simulink model "OpenLoopTest_animacion"  (R2023a)
settings: Solver=VariableStepAuto  StartTime=0.0  StopTime=50  RelTol=1e-3
model workspace (MAT data in the model file):
  A = 0.000165129963854
  B = 2.18020469989e-05
  I = [0.0336109715  0  0; 0  0.0308250765  0; 0  0  0.0271714972]
  Iw = [7.613e-05  0  0; 0  7.613e-05  0; 0  0  7.613e-05]
  J = 7.613e-05
  Ke = 0.00852615766564
  Kt = 0.00855
  L = 0.585
  La = 0.000222
  Ra = 3.36
  T_ext = 6.85e-07
  T_max = 7.7501
  T_max_mgt = -0.018432
  coil_longitude = 7.92
  dia_coil = 2
  dia_core = 0.77
  dia_wire = 0.03
  l = 0.0792
  mu_0 = 1.25663706212e-06
  mu_r = 200000
  n = 33.4123983836
  n_cal = 5412
  n_layers = 20.5
  s = tf
  s.IOSize_ = [1 1]
  s.Data_ = ltipack.tfdata
  s.Data_.num = {[1 0]}
  s.Data_.den = {[0 1]}
  s.Data_.Delay.Input = 0
  s.Data_.Delay.Output = 0
  s.Data_.Delay.IO = 0
  s.Data_.Ts = 0
  sys = tf
  sys.IOSize_ = [1 1]
  sys.Data_ = ltipack.tfdata
  sys.Data_.num = {[0 6.509115e-07 1.86407501841e-07]}
  sys.Data_.den = {[1.690086e-08 0.000255801640054 0.000146153525957]}
  sys.Data_.Delay.Input = 0
  sys.Data_.Delay.Output = 0
  sys.Data_.Delay.IO = 0
  sys.Data_.Ts = 0
  turns_per_layer = 264
  voltaje = 9
libraries: simulink_extras x6, aerolibutil x2, vrlib x1, shared6dofsys x1
settings Model: Creator=Personal  LastModifiedBy=Personal
settings OptimizationCC: ReuseModelBlockBuffer=off

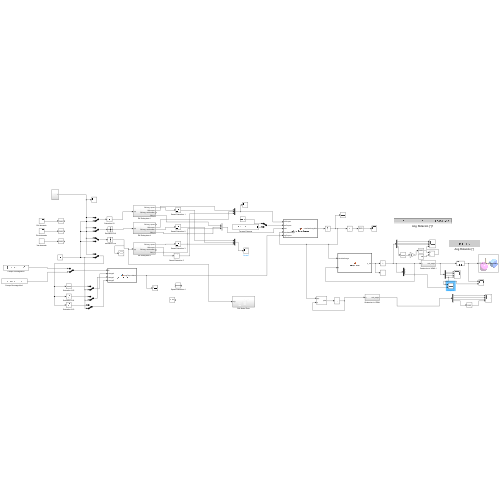
[thumbnail: Simulink's stored preview of the top-level diagram]
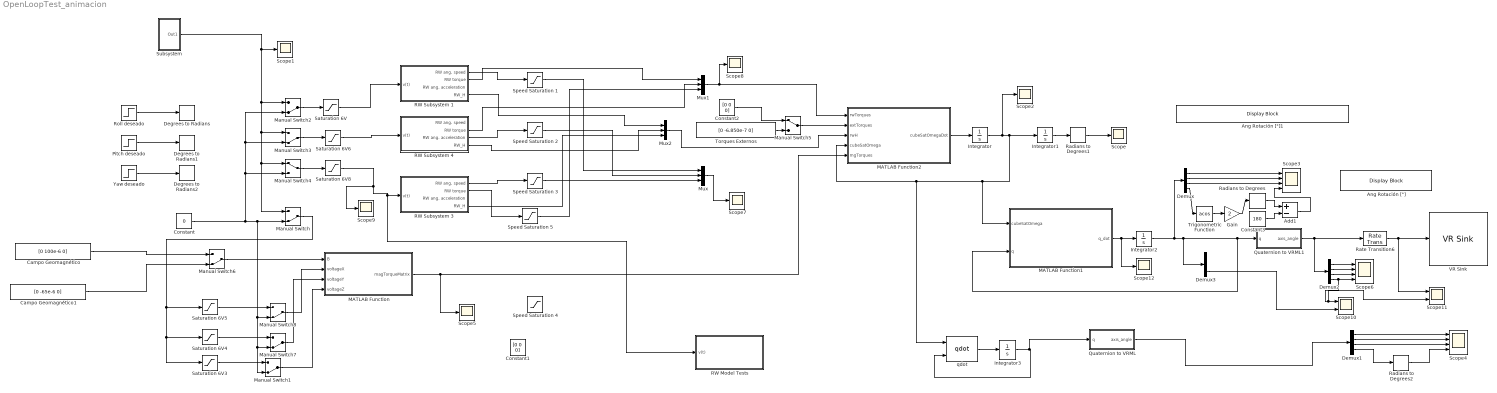
== system OpenLoopTest_animacion ==
  Add1 : Sum  Inputs=+-
  Ang Rotación [°] : DisplayBlock  LabelPosition=Hide  Transparency=1
  Ang Rotación [°]1 : DisplayBlock  LabelPosition=Hide  Transparency=1
  Campo Geomagnético : Constant  Value=[0 100e-6 0]
  Campo Geomagnético1 : Constant  Value=[0 -65e-6 0]
  Constant : Constant  Value=0
  Constant1 : Constant  Value=[0 0 0]
  Constant2 : Constant  Value=[0 0 0]
  Constant3 : Constant  Value=180
  Degrees to Radians : simulink_extras/Transformations/Degrees to Radians
  Degrees to Radians1 : simulink_extras/Transformations/Degrees to Radians
  Degrees to Radians2 : simulink_extras/Transformations/Degrees to Radians
  Demux{,1..3} (4 alike) : Demux
  Gain : Gain  Gain=2
  Integrator : Integrator  InitialCondition=[0 0 0]
  Integrator1 : Integrator  InitialCondition=[0 0 0]
  Integrator2 : Integrator  InitialCondition=[0 0 1 0]
  Integrator3 : Integrator  InitialCondition=[0 1 0 0]
  MATLAB Function : MATLAB Function  TreatAsAtomicUnit=on
  MATLAB Function1 : MATLAB Function  TreatAsAtomicUnit=on
  MATLAB Function2 : MATLAB Function  TreatAsAtomicUnit=on
  Manual Switch{,1..3,6..8} (7 alike) : ManualSwitch  CurrentSetting=0
  Manual Switch4 : ManualSwitch
  Manual Switch5 : ManualSwitch
  Mux : Mux  Inputs=3
  Mux1 : Mux  Inputs=3
  Mux2 : Mux  Inputs=3
  Pitch deseado : Step  Time=2  After=0  SampleTime=0
  Quaternion to VRML : Subsystem
  Quaternion to VRML1 : Subsystem
  RW Model Tests : Subsystem
  RW Subsystem 1 : Subsystem
  RW Subsystem 3 : Subsystem
  RW Subsystem 4 : Subsystem
  Radians to Degrees : simulink_extras/Transformations/Radians to Degrees
  Radians to Degrees1 : simulink_extras/Transformations/Radians to Degrees
  Radians to Degrees2 : simulink_extras/Transformations/Radians to Degrees
  Rate Transition6 : RateTransition
  Roll deseado : Step  Time=2  After=90  SampleTime=0
  Saturation 6V : Saturate  UpperLimit=5  LowerLimit=-5
  Saturation 6V3 : Saturate  UpperLimit=6  LowerLimit=-6
  Saturation 6V4 : Saturate  UpperLimit=2  LowerLimit=-6
  Saturation 6V5 : Saturate  UpperLimit=5  LowerLimit=-5
  Saturation 6V6 : Saturate  UpperLimit=5  LowerLimit=-5
  Saturation 6V8 : Saturate  UpperLimit=6  LowerLimit=0
  Scope{,1..2,5,7..9,12} (8 alike) : Scope
  Scope10 : Scope  NumInputPorts=2
  Scope11 : Scope  NumInputPorts=2
  Scope3 : Scope  NumInputPorts=4
  Scope4 : Scope  NumInputPorts=4
  Scope6 : Scope  NumInputPorts=4
  Speed Saturation {1..5} (5 alike) : Saturate  UpperLimit=8000  LowerLimit=0
  Subsystem : Subsystem
  Torques Externos : Constant  Value=[0 -6.850e-7 0]
  Trigonometric Function : Trigonometry  Operator=acos
  VR Sink : vrlib/VR Sink  InstantiateOnLoad=on  SampleTime=0.1  ViewEnable=on  RemoteChange=off  RemoteView=off  FieldsWritten=STLB_Transform.rotation.4.1.1.double  WorldFileName=EscenarioCubeSat.x3d  AutoView=off  VideoDimensions=[]  AllowVariableSize=off
  Yaw deseado : Step  Time=2  After=180  SampleTime=0
  qdot : shared6dofsys/qdot  aMode=aMode
  wires:
  Roll deseado/1 -> Degrees to Radians/1
  Yaw deseado/1 -> Degrees to Radians2/1
  Pitch deseado/1 -> Degrees to Radians1/1
  Saturation 6V/1 -> RW Subsystem 1/1(v(t))
  Saturation 6V6/1 -> RW Subsystem 4/1(v(t))
  Saturation 6V8/1 -> Scope9/1, RW Model Tests/1(v(t)), RW Subsystem 3/1(v(t))
  RW Subsystem 3/1(RW ang. speed) -> Speed Saturation 3/1
  Speed Saturation 1/1 -> Mux/1
  Speed Saturation 2/1 -> Mux/2
  Speed Saturation 3/1 -> Mux/3
  MATLAB Function2/1(cubeSatOmegaDot) -> Integrator/1
  Integrator/1 -> Scope2/1, Integrator1/1, MATLAB Function1/1(cubeSatOmega), qdot/1, MATLAB Function2/4(cubeSatOmega)
  Integrator1/1 -> Radians to Degrees1/1
  Mux/1 -> Scope7/1
  Mux1/1 -> Scope8/1, MATLAB Function2/1(rwTorques)
  MATLAB Function/1(magTorqueMatrix) -> Scope5/1, MATLAB Function2/5(mgTorques)
  Constant/1 -> Manual Switch2/2, Manual Switch3/2, Manual Switch4/2, Manual Switch1/2, Manual Switch7/2, Manual Switch8/2, Manual Switch/2
  Manual Switch/1 -> Saturation 6V4/1, Saturation 6V3/1, Saturation 6V5/1
  Saturation 6V3/1 -> Manual Switch1/1
  Manual Switch1/1 -> MATLAB Function/4(voltageZ)
  Manual Switch2/1 -> Saturation 6V/1
  Manual Switch3/1 -> Saturation 6V6/1
  Manual Switch4/1 -> Saturation 6V8/1
  Torques Externos/1 -> Manual Switch5/2
  Manual Switch5/1 -> MATLAB Function2/2(extTorques)
  Constant2/1 -> Manual Switch5/1
  Manual Switch6/1 -> MATLAB Function/1(B)
  Campo Geomagnético/1 -> Manual Switch6/1
  Campo Geomagnético1/1 -> Manual Switch6/2
  Saturation 6V4/1 -> Manual Switch7/1
  Saturation 6V5/1 -> Manual Switch8/1
  Manual Switch8/1 -> MATLAB Function/2(voltageX)
  Manual Switch7/1 -> MATLAB Function/3(voltageY)
  MATLAB Function1/1(q_dot) -> Scope12/1, Integrator2/1
  Integrator2/1 -> Demux/1, Demux3/1, Quaternion to VRML1/1(q), MATLAB Function1/2(q)
  Demux/1 -> Scope3/1
  Demux/2 -> Scope3/2
  Demux/3 -> Scope3/3
  Radians to Degrees/1 -> Add1/1
  Radians to Degrees1/1 -> Scope/1
  Rate Transition6/1 -> Scope11/1, VR Sink/1
  Radians to Degrees2/1 -> Scope4/4
  Demux1/4 -> Radians to Degrees2/1
  Demux1/3 -> Scope4/3
  Demux1/2 -> Scope4/2
  Demux1/1 -> Scope4/1
  Quaternion to VRML/1(axis_angle) -> Demux1/1
  Demux/4 -> Trigonometric Function/1
  Trigonometric Function/1 -> Gain/1
  Gain/1 -> Radians to Degrees/1
  Demux2/1 -> Scope6/1
  Demux2/2 -> Scope6/2
  Demux2/3 -> Scope6/3
  Demux2/4 -> Scope11/2, Scope10/1, Scope6/4
  qdot/1 -> Integrator3/1
  Integrator3/1 -> Quaternion to VRML/1(q), qdot/2
  Quaternion to VRML1/1(axis_angle) -> Demux2/1, Rate Transition6/1
  Constant3/1 -> Add1/2
  Add1/1 -> Scope3/4
  RW Subsystem 3/2(RW torque) -> Speed Saturation 5/1
  Speed Saturation 5/1 -> Mux1/3
  Demux3/4 -> Scope10/2
  RW Subsystem 1/1(RW ang. speed) -> Speed Saturation 1/1
  RW Subsystem 1/2(RW torque) -> Mux1/1
  RW Subsystem 4/3(RW ang. acceleration) -> Speed Saturation 2/1
  RW Subsystem 4/2(RW torque) -> Mux1/2
  RW Subsystem 4/4(RW_H) -> Mux2/2
  RW Subsystem 3/4(RW_H) -> Mux2/3
  RW Subsystem 1/4(RW_H) -> Mux2/1
  Mux2/1 -> MATLAB Function2/3(rwH)
  Subsystem/1(Out1) -> Manual Switch2/1, Manual Switch3/1, Manual Switch4/1, Manual Switch/1, Scope1/1

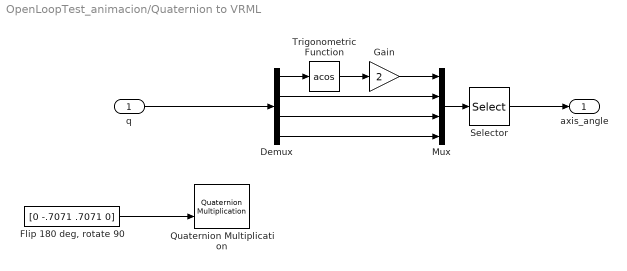
== system OpenLoopTest_animacion/Quaternion to VRML ==
  q : Inport
  Demux : Demux
  "Flip 180 deg, rotate 90" : Constant  Value=[0 -.7071 .7071 0]
  Gain : Gain  Gain=2
  Mux : Mux
  Quaternion Multiplication : aerolibutil/Quaternion Multiplication
  Selector : Selector  InputPortWidth=4  IndexOptions=Index vector (dialog)  Indices=[3 4 2 1]  OutputSizes=1
  Trigonometric Function : Trigonometry  Operator=acos
  axis_angle : Outport  VectorParamsAs1DForOutWhenUnconnected=off
  wires:
  Demux/4 -> Mux/4
  Gain/1 -> Mux/1
  Selector/1 -> axis_angle/1
  q/1 -> Demux/1
  Mux/1 -> Selector/1
  Trigonometric Function/1 -> Gain/1
  Demux/1 -> Trigonometric Function/1
  "Flip 180 deg, rotate 90"/1 -> Quaternion Multiplication/2
  Demux/2 -> Mux/2
  Demux/3 -> Mux/3

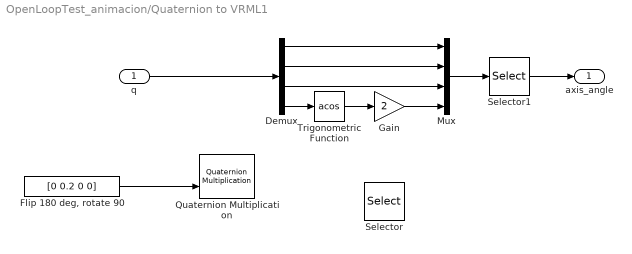
== system OpenLoopTest_animacion/Quaternion to VRML1 ==
  q : Inport
  Demux : Demux
  "Flip 180 deg, rotate 90" : Constant  Value=[0 0.2 0 0]
  Gain : Gain  Gain=2
  Mux : Mux
  Quaternion Multiplication : aerolibutil/Quaternion Multiplication
  Selector : Selector  InputPortWidth=3  IndexOptions=Index vector (dialog)  Indices=[1 3]  OutputSizes=1
  Selector1 : Selector  InputPortWidth=4  IndexOptions=Index vector (dialog)  Indices=[2 3 1 4]  OutputSizes=1
  Trigonometric Function : Trigonometry  Operator=acos
  axis_angle : Outport  VectorParamsAs1DForOutWhenUnconnected=off
  wires:
  Demux/3 -> Mux/3
  Demux/2 -> Mux/2
  "Flip 180 deg, rotate 90"/1 -> Quaternion Multiplication/2
  Trigonometric Function/1 -> Gain/1
  q/1 -> Demux/1
  Gain/1 -> Mux/4
  Demux/4 -> Trigonometric Function/1
  Demux/1 -> Mux/1
  Mux/1 -> Selector1/1
  Selector1/1 -> axis_angle/1

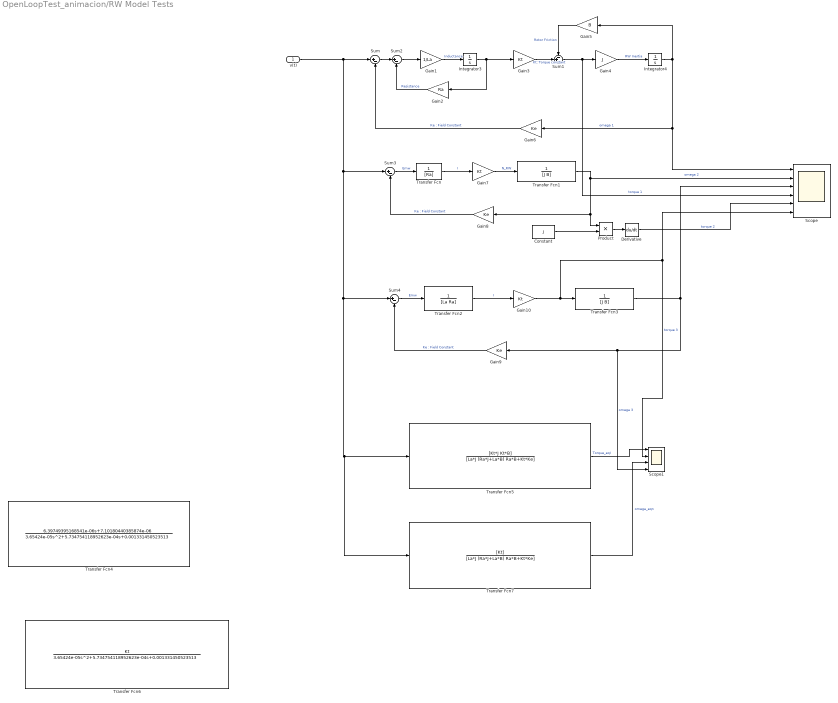
== system OpenLoopTest_animacion/RW Model Tests ==
  v(t) : Inport
  Constant : Constant  Value=J
  Derivative : Derivative
  Gain1 : Gain  Gain=1/La
  Gain10 : Gain  Gain=Kt
  Gain2 : Gain  Gain=Ra
  Gain3 : Gain  Gain=Kt
  Gain4 : Gain  Gain=J
  Gain5 : Gain  Gain=B
  Gain6 : Gain  Gain=Ke
  Gain7 : Gain  Gain=Kt
  Gain8 : Gain  Gain=Ke
  Gain9 : Gain  Gain=Ke
  Integrator3 : Integrator
  Integrator4 : Integrator
  Product : Product
  Scope : Scope  NumInputPorts=6
  Scope1 : Scope  NumInputPorts=4
  Sum{,2..4} (4 alike) : Sum  Inputs=|+-
  Sum1 : Sum  Inputs=-+|
  Transfer Fcn : TransferFcn  Denominator=[Ra]
  Transfer Fcn1 : TransferFcn  Denominator=[J B]
  Transfer Fcn2 : TransferFcn  Denominator=[La Ra]
  Transfer Fcn3 : TransferFcn  Denominator=[J B]
  Transfer Fcn4 : TransferFcn  Numerator=[6.39749395168541e-06 7.10180440385874e-06]  Denominator=[3.65424e-05 5.734754118952623e-04 0.001331450523513]
  Transfer Fcn5 : TransferFcn  Numerator=[Kt*J Kt*B]  Denominator=[La*J (Ra*J+La*B) Ra*B+Kt*Ke]
  Transfer Fcn6 : TransferFcn  Numerator=Kt  Denominator=[3.65424e-05 5.734754118952623e-04 0.001331450523513]
  Transfer Fcn7 : TransferFcn  Numerator=[Kt]  Denominator=[La*J (Ra*J+La*B) Ra*B+Kt*Ke]
  wires:
  Sum1/1 -> Gain4/1, Scope/4  "torque 1"
  Derivative/1 -> Scope/5  "torque 2"
  Transfer Fcn3/1 -> Scope/3, Gain9/1, Scope1/4  "omega 3"
  Gain10/1 -> Transfer Fcn3/1, Scope/6, Scope1/2  "torque 3"
  Transfer Fcn2/1 -> Gain10/1  "I"
  Gain9/1 -> Sum4/2  "Ke : Field Constant"
  Sum4/1 -> Transfer Fcn2/1  "Emw"
  Gain2/1 -> Sum2/2  "Resistance"
  Integrator3/1 -> Gain2/1, Gain3/1
  Gain6/1 -> Sum/2  "Ke : Field Constant"
  Gain5/1 -> Sum1/1  "Rotor Friction"
  Sum2/1 -> Gain1/1
  Integrator4/1 -> Gain6/1, Scope/1, Gain5/1  "omega 1"
  Gain4/1 -> Integrator4/1  "RW Inertia"
  Gain1/1 -> Integrator3/1  "Inductance"
  Gain3/1 -> Sum1/2  "Kt: Torque constant"
  Sum/1 -> Sum2/1
  v(t)/1 -> Transfer Fcn7/1, Transfer Fcn5/1, Sum4/1, Sum3/1, Sum/1
  Sum3/1 -> Transfer Fcn/1  "Emw"
  Gain7/1 -> Transfer Fcn1/1  "N_RW"
  Transfer Fcn/1 -> Gain7/1  "I"
  Transfer Fcn1/1 -> Product/1, Gain8/1, Scope/2  "omega 2"
  Gain8/1 -> Sum3/2  "Ke : Field Constant"
  Product/1 -> Derivative/1
  Constant/1 -> Product/2
  Transfer Fcn5/1 -> Scope1/1  "Torque_eqI"
  Transfer Fcn7/1 -> Scope1/3  "omega_eqn"

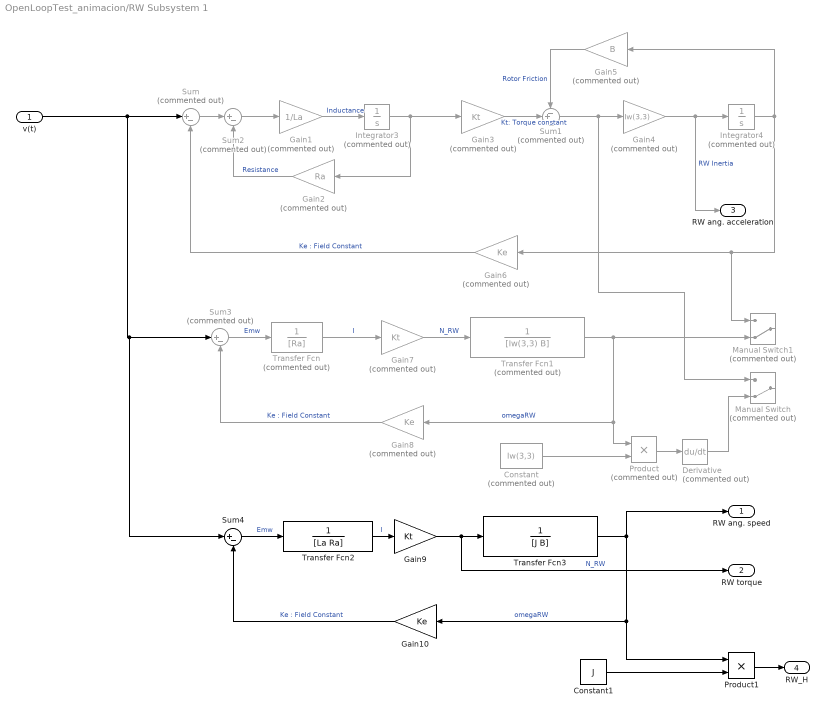
== system OpenLoopTest_animacion/RW Subsystem 1 ==
  v(t) : Inport
  Constant : Constant  Commented=on  Value=Iw(3,3)
  Constant1 : Constant  Value=J
  Derivative : Derivative  Commented=on
  Gain1 : Gain  Commented=on  Gain=1/La
  Gain10 : Gain  Gain=Ke
  Gain2 : Gain  Commented=on  Gain=Ra
  Gain3 : Gain  Commented=on  Gain=Kt
  Gain4 : Gain  Commented=on  Gain=Iw(3,3)
  Gain5 : Gain  Commented=on  Gain=B
  Gain6 : Gain  Commented=on  Gain=Ke
  Gain7 : Gain  Commented=on  Gain=Kt
  Gain8 : Gain  Commented=on  Gain=Ke
  Gain9 : Gain  Gain=Kt
  Integrator3 : Integrator  Commented=on
  Integrator4 : Integrator  Commented=on
  Manual Switch : ManualSwitch  Commented=on  CurrentSetting=0
  Manual Switch1 : ManualSwitch  Commented=on  CurrentSetting=0
  Product : Product  Commented=on
  Product1 : Product
  Sum : Sum  Commented=on  Inputs=|+-
  Sum1 : Sum  Commented=on  Inputs=-+|
  Sum2 : Sum  Commented=on  Inputs=|+-
  Sum3 : Sum  Commented=on  Inputs=|+-
  Sum4 : Sum  Inputs=|+-
  Transfer Fcn : TransferFcn  Commented=on  Denominator=[Ra]
  Transfer Fcn1 : TransferFcn  Commented=on  Denominator=[Iw(3,3) B]
  Transfer Fcn2 : TransferFcn  Denominator=[La Ra]
  Transfer Fcn3 : TransferFcn  Denominator=[J B]
  RW ang. speed : Outport  VectorParamsAs1DForOutWhenUnconnected=off
  RW torque : Outport  Port=2  VectorParamsAs1DForOutWhenUnconnected=off
  RW ang. acceleration : Outport  Port=3  VectorParamsAs1DForOutWhenUnconnected=off
  RW_H : Outport  Port=4  VectorParamsAs1DForOutWhenUnconnected=off
  wires:
  Gain2/1 -> Sum2/2  "Resistance"
  Integrator3/1 -> Gain2/1, Gain3/1
  Gain6/1 -> Sum/2  "Ke : Field Constant"
  Gain5/1 -> Sum1/1  "Rotor Friction"
  Sum2/1 -> Gain1/1
  Sum1/1 -> Gain4/1, Manual Switch/1
  Integrator4/1 -> Manual Switch1/1, Gain6/1, Gain5/1
  Gain4/1 -> Integrator4/1, RW ang. acceleration/1  "RW Inertia"
  Gain1/1 -> Integrator3/1  "Inductance"
  Gain3/1 -> Sum1/2  "Kt: Torque constant"
  Sum/1 -> Sum2/1
  Sum3/1 -> Transfer Fcn/1  "Emw"
  Gain7/1 -> Transfer Fcn1/1  "N_RW"
  Transfer Fcn/1 -> Gain7/1  "I"
  Transfer Fcn1/1 -> Product/1, Gain8/1, Manual Switch1/2  "omegaRW"
  Gain8/1 -> Sum3/2  "Ke : Field Constant"
  Product/1 -> Derivative/1
  Constant/1 -> Product/2
  Derivative/1 -> Manual Switch/2
  Gain10/1 -> Sum4/2  "Ke : Field Constant"
  Transfer Fcn3/1 -> Product1/1, Gain10/1, RW ang. speed/1  "omegaRW"
  Transfer Fcn2/1 -> Gain9/1  "I"
  Gain9/1 -> RW torque/1, Transfer Fcn3/1  "N_RW"
  Sum4/1 -> Transfer Fcn2/1  "Emw"
  v(t)/1 -> Sum4/1, Sum3/1, Sum/1
  Constant1/1 -> Product1/2
  Product1/1 -> RW_H/1

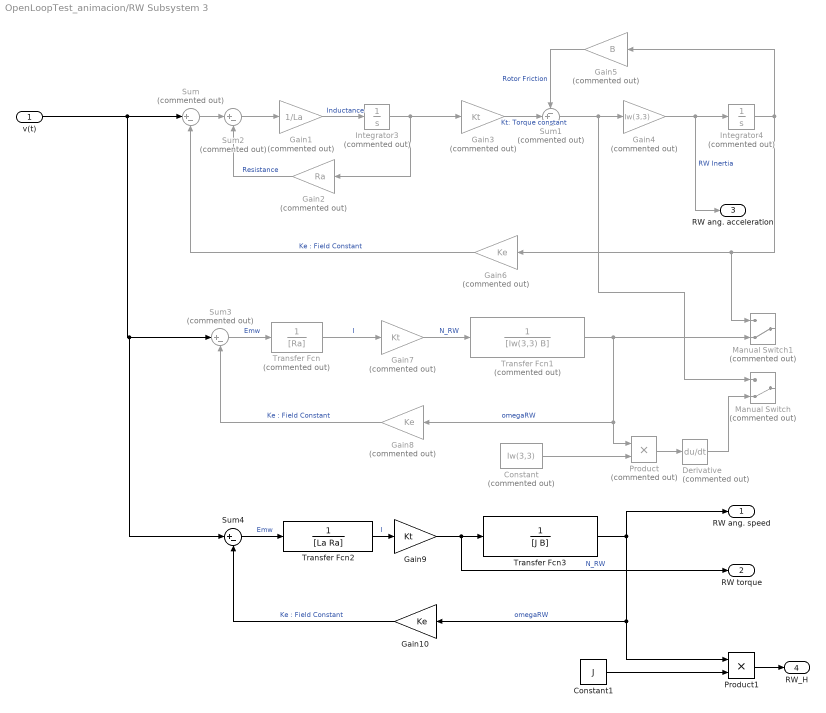
== system OpenLoopTest_animacion/RW Subsystem 3 ==
  v(t) : Inport
  Constant : Constant  Commented=on  Value=Iw(3,3)
  Constant1 : Constant  Value=J
  Derivative : Derivative  Commented=on
  Gain1 : Gain  Commented=on  Gain=1/La
  Gain10 : Gain  Gain=Ke
  Gain2 : Gain  Commented=on  Gain=Ra
  Gain3 : Gain  Commented=on  Gain=Kt
  Gain4 : Gain  Commented=on  Gain=Iw(3,3)
  Gain5 : Gain  Commented=on  Gain=B
  Gain6 : Gain  Commented=on  Gain=Ke
  Gain7 : Gain  Commented=on  Gain=Kt
  Gain8 : Gain  Commented=on  Gain=Ke
  Gain9 : Gain  Gain=Kt
  Integrator3 : Integrator  Commented=on
  Integrator4 : Integrator  Commented=on
  Manual Switch : ManualSwitch  Commented=on  CurrentSetting=0
  Manual Switch1 : ManualSwitch  Commented=on  CurrentSetting=0
  Product : Product  Commented=on
  Product1 : Product
  Sum : Sum  Commented=on  Inputs=|+-
  Sum1 : Sum  Commented=on  Inputs=-+|
  Sum2 : Sum  Commented=on  Inputs=|+-
  Sum3 : Sum  Commented=on  Inputs=|+-
  Sum4 : Sum  Inputs=|+-
  Transfer Fcn : TransferFcn  Commented=on  Denominator=[Ra]
  Transfer Fcn1 : TransferFcn  Commented=on  Denominator=[Iw(3,3) B]
  Transfer Fcn2 : TransferFcn  Denominator=[La Ra]
  Transfer Fcn3 : TransferFcn  Denominator=[J B]
  RW ang. speed : Outport  VectorParamsAs1DForOutWhenUnconnected=off
  RW torque : Outport  Port=2  VectorParamsAs1DForOutWhenUnconnected=off
  RW ang. acceleration : Outport  Port=3  VectorParamsAs1DForOutWhenUnconnected=off
  RW_H : Outport  Port=4  VectorParamsAs1DForOutWhenUnconnected=off
  wires:
  Gain2/1 -> Sum2/2  "Resistance"
  Integrator3/1 -> Gain2/1, Gain3/1
  Gain6/1 -> Sum/2  "Ke : Field Constant"
  Gain5/1 -> Sum1/1  "Rotor Friction"
  Sum2/1 -> Gain1/1
  Sum1/1 -> Gain4/1, Manual Switch/1
  Integrator4/1 -> Manual Switch1/1, Gain6/1, Gain5/1
  Gain4/1 -> Integrator4/1, RW ang. acceleration/1  "RW Inertia"
  Gain1/1 -> Integrator3/1  "Inductance"
  Gain3/1 -> Sum1/2  "Kt: Torque constant"
  Sum/1 -> Sum2/1
  Sum3/1 -> Transfer Fcn/1  "Emw"
  Gain7/1 -> Transfer Fcn1/1  "N_RW"
  Transfer Fcn/1 -> Gain7/1  "I"
  Transfer Fcn1/1 -> Product/1, Gain8/1, Manual Switch1/2  "omegaRW"
  Gain8/1 -> Sum3/2  "Ke : Field Constant"
  Product/1 -> Derivative/1
  Constant/1 -> Product/2
  Derivative/1 -> Manual Switch/2
  Gain10/1 -> Sum4/2  "Ke : Field Constant"
  Transfer Fcn3/1 -> Product1/1, Gain10/1, RW ang. speed/1  "omegaRW"
  Transfer Fcn2/1 -> Gain9/1  "I"
  Gain9/1 -> RW torque/1, Transfer Fcn3/1  "N_RW"
  Sum4/1 -> Transfer Fcn2/1  "Emw"
  v(t)/1 -> Sum4/1, Sum3/1, Sum/1
  Constant1/1 -> Product1/2
  Product1/1 -> RW_H/1

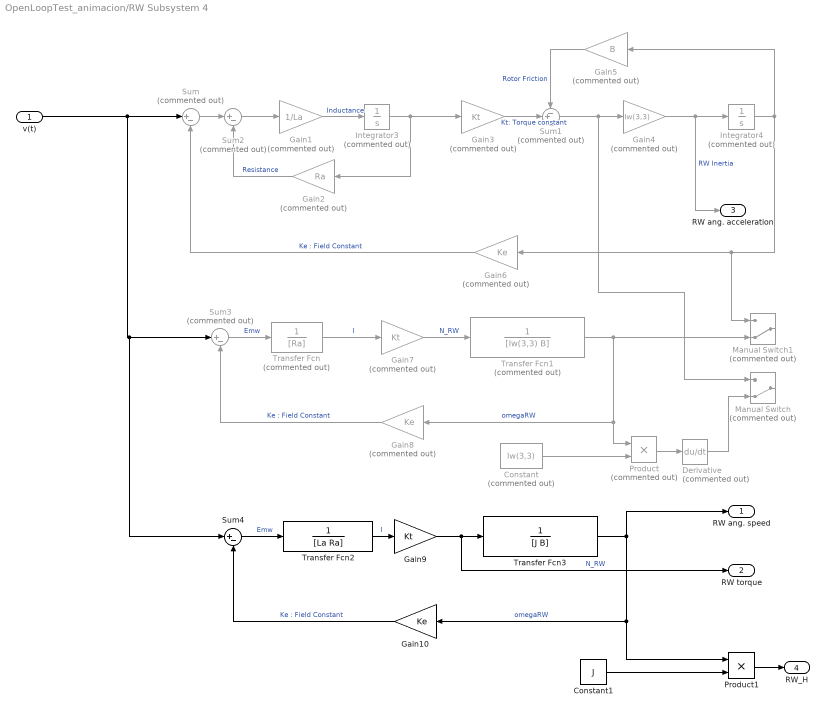
== system OpenLoopTest_animacion/RW Subsystem 4 ==
  v(t) : Inport
  Constant : Constant  Commented=on  Value=Iw(3,3)
  Constant1 : Constant  Value=J
  Derivative : Derivative  Commented=on
  Gain1 : Gain  Commented=on  Gain=1/La
  Gain10 : Gain  Gain=Ke
  Gain2 : Gain  Commented=on  Gain=Ra
  Gain3 : Gain  Commented=on  Gain=Kt
  Gain4 : Gain  Commented=on  Gain=Iw(3,3)
  Gain5 : Gain  Commented=on  Gain=B
  Gain6 : Gain  Commented=on  Gain=Ke
  Gain7 : Gain  Commented=on  Gain=Kt
  Gain8 : Gain  Commented=on  Gain=Ke
  Gain9 : Gain  Gain=Kt
  Integrator3 : Integrator  Commented=on
  Integrator4 : Integrator  Commented=on
  Manual Switch : ManualSwitch  Commented=on  CurrentSetting=0
  Manual Switch1 : ManualSwitch  Commented=on  CurrentSetting=0
  Product : Product  Commented=on
  Product1 : Product
  Sum : Sum  Commented=on  Inputs=|+-
  Sum1 : Sum  Commented=on  Inputs=-+|
  Sum2 : Sum  Commented=on  Inputs=|+-
  Sum3 : Sum  Commented=on  Inputs=|+-
  Sum4 : Sum  Inputs=|+-
  Transfer Fcn : TransferFcn  Commented=on  Denominator=[Ra]
  Transfer Fcn1 : TransferFcn  Commented=on  Denominator=[Iw(3,3) B]
  Transfer Fcn2 : TransferFcn  Denominator=[La Ra]
  Transfer Fcn3 : TransferFcn  Denominator=[J B]
  RW ang. speed : Outport  VectorParamsAs1DForOutWhenUnconnected=off
  RW torque : Outport  Port=2  VectorParamsAs1DForOutWhenUnconnected=off
  RW ang. acceleration : Outport  Port=3  VectorParamsAs1DForOutWhenUnconnected=off
  RW_H : Outport  Port=4  VectorParamsAs1DForOutWhenUnconnected=off
  wires:
  Product1/1 -> RW_H/1
  Constant1/1 -> Product1/2
  v(t)/1 -> Sum/1, Sum3/1, Sum4/1
  Sum4/1 -> Transfer Fcn2/1  "Emw"
  Gain9/1 -> Transfer Fcn3/1, RW torque/1  "N_RW"
  Transfer Fcn2/1 -> Gain9/1  "I"
  Transfer Fcn3/1 -> RW ang. speed/1, Gain10/1, Product1/1  "omegaRW"
  Gain10/1 -> Sum4/2  "Ke : Field Constant"
  Derivative/1 -> Manual Switch/2
  Constant/1 -> Product/2
  Product/1 -> Derivative/1
  Gain8/1 -> Sum3/2  "Ke : Field Constant"
  Transfer Fcn1/1 -> Manual Switch1/2, Gain8/1, Product/1  "omegaRW"
  Transfer Fcn/1 -> Gain7/1  "I"
  Gain7/1 -> Transfer Fcn1/1  "N_RW"
  Sum3/1 -> Transfer Fcn/1  "Emw"
  Sum/1 -> Sum2/1
  Gain3/1 -> Sum1/2  "Kt: Torque constant"
  Gain1/1 -> Integrator3/1  "Inductance"
  Gain4/1 -> RW ang. acceleration/1, Integrator4/1  "RW Inertia"
  Integrator4/1 -> Gain5/1, Gain6/1, Manual Switch1/1
  Sum1/1 -> Manual Switch/1, Gain4/1
  Sum2/1 -> Gain1/1
  Gain5/1 -> Sum1/1  "Rotor Friction"
  Gain6/1 -> Sum/2  "Ke : Field Constant"
  Integrator3/1 -> Gain3/1, Gain2/1
  Gain2/1 -> Sum2/2  "Resistance"

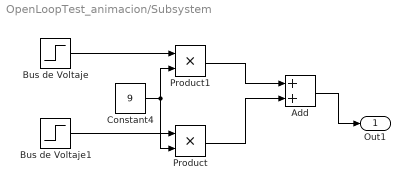
== system OpenLoopTest_animacion/Subsystem ==
  Add : Sum
  Bus de Voltaje : Step  Time=3  SampleTime=0
  Bus de Voltaje1 : Step  Time=5  After=-1  SampleTime=0
  Constant4 : Constant  Value=9
  Product : Product
  Product1 : Product
  Out1 : Outport
  wires:
  Product/1 -> Add/2
  Add/1 -> Out1/1
  Constant4/1 -> Product/2, Product1/2
  Bus de Voltaje1/1 -> Product/1
  Product1/1 -> Add/1
  Bus de Voltaje/1 -> Product1/1

== matlab function OpenLoopTest_animacion/MATLAB Function1 ==
  data: cubeSatOmega input; q_dot output; q input
function q_dot = omega2qdot(cubeSatOmega,q)

wx = cubeSatOmega(1);
wy = cubeSatOmega(2);
wz = cubeSatOmega(3);

OmegaMatrix = [0 wz -wy wx ;
               -wz 0 wx wy; 
               wy -wx 0 wz;
               -wx -wy -wz 0];
            
q_dot=0.5*OmegaMatrix*q;

end

== matlab function OpenLoopTest_animacion/MATLAB Function ==
  data: B input; magTorqueMatrix output; voltageX input; voltageY input; voltageZ input
function magTorqueMatrix = magTorqueFunction(B,voltageX,voltageY,voltageZ)

d = 1.45e-2; % Diametro mgt [m]
A =d^2*pi/4;
%A =10;
mu_0 = 1.25663706212e-12; % Permeabilidad del vacío [Vs/Am]
mu_r = 200000; % Permeabilidad del relativa del Hierro [-] Ref-> http://hyperphysics.phy-astr.gsu.edu/hbase/Tables/magprop.html#c2
%L = 0.585; % H % Impedancia [H] 
L = 11.2534e-3; % Impedancia [H] 
l = 7.92e-2; % Longitud mgt [m] 

n=sqrt(L*l/(mu_0*mu_r*A)); % # Vueltas 

R = 50.7 ;% Resistencia mgt [Ohm];
ix = voltageX/R;
iy = voltageY/R;
iz = voltageZ/R;




magTorqueMatrix_X = cross(n*ix*A*[1 0 0],B);
magTorqueMatrix_Y = cross(n*iy*A*[0 1 0],B);
magTorqueMatrix_Z = cross(n*iz*A*[0 0 1],B);


magTorqueMatrix = magTorqueMatrix_X+magTorqueMatrix_Y+magTorqueMatrix_Z;

== matlab function OpenLoopTest_animacion/MATLAB Function2 ==
  data: rwTorques input; cubeSatOmegaDot output; extTorques input; rwH input; cubeSatOmega input; mgTorques input
function cubeSatOmegaDot = cubeSatDynamicModel(rwTorques,extTorques,rwH,cubeSatOmega,mgTorques)

% Inercia EyasSat [kg m2]
I =1e-7*[336109.715 0 0 ;
        0 308250.765 0; 
        0 0 271714.972];

% % Inercia EyasSat [kg m2]
% I =1e-7*[335592.028 0 0 ;
%         0 335592.028 0; 
%         0 0 335592.028];

%Momentos de inercia EyasSat
Ixx = I(1,1);
Iyy = I(2,2);
Izz = I(3,3);





% % Inercia RW [kg m2]
% Iw = 1e-5*[1 0 0 ;
%            0 1 0 ;
%            0 0 1 ]; %kg m2

%Momento angular RW


%Velocidades angulares EyasSat
wx = cubeSatOmega(1);
wy = cubeSatOmega(2);
wz = cubeSatOmega(3);

%Torques externos
Tx = extTorques(1);
Ty = extTorques(2);
Tz = extTorques(3);

%Torques de control RW
Tc_x = rwTorques(1);
Tc_y = rwTorques(2);
Tc_z = rwTorques(3);

%Torques de control RW
Tmg_x = mgTorques(1);
Tmg_y = mgTorques(2);
Tmg_z = mgTorques(3);

hx = rwH(1);
hy = rwH(2);
hz = rwH(3);



omegaDotX = (Tx+Tc_x+Tmg_x+wy*wz*(Iyy-Izz)-hz*wy+hy*wz)/Ixx;
omegaDotY = (Ty+Tc_y+Tmg_y+wx*wz*(Izz-Ixx)-hx*wz+hz*wx)/Iyy;
omegaDotZ = (Tz+Tc_z+Tmg_z+wx*wy*(Ixx-Iyy)-hy*wx+hx*wy)/Izz;

cubeSatOmegaDot = [omegaDotX omegaDotY omegaDotZ];
